simulink model "lht_workflow"  (R2020a)
settings: Solver=FixedStepDiscrete  StartTime=0.0  StopTime=inf  RelTol=1e-3
InitFcn:
  | % Clear workspace
  | clc; clear; close all;
  | 
  | % Set parameters
  | height = 240;
  | width = 320;
  | sobelThreshold = 30;
  | dTheta = 1;
  | dRho = 1;
  | 
  | % Read in image and resize
  | I = imread('roof.bmp');
  | Ir = imresize(I, [height, width]);
  | 
  | % Get greyscale
  | Y = rgb2gray(Ir);
  | 
  | % Get Edge and Gradient Orientation image
  | [edge] = Sobel(Y, sobelThreshold);
  | 
  | % Create input array
  | inarray = uint8(fi(edge, 0, 1, 0));
  | 
  | hdlset_param(gcs, 'GenerateValidationModel', 'on');
  | 
  | % Memory
  | maxRho = ceil(sqrt((height/2)^2+(width/2)^2));
  | bitsRho = ceil(log2(maxRho*2));
StopFcn:
  | %Get theta and rho
  | theta = 0:dTheta:180-dTheta;
  | 
  | A = reshape(out.simout, [maxRho*2, numel(theta)]);
  | 
  | plot3DHPS(A);
libraries: hdlsllib x5, simulink x2, dspsrcs4 x1
settings Model: DataTypeOverride=Off  SimulationMode=accelerator  Creator=david  LastModifiedBy=david
settings DataIOCC: SaveOutput=off  SaveTime=off
settings OptimizationCC: BlockReduction=off  ConditionallyExecuteInputs=off  DefaultParameterBehavior=Inlined
settings DebuggingCC: AlgebraicLoopMsg=error  SingleTaskRateTransMsg=error
settings HardwareCC: ProdBitPerPointer=32  ProdBitPerSizeT=32  ProdBitPerPtrDiffT=32  ProdLargestAtomicFloat=None  ProdIntDivRoundTo=Undefined  ProdEndianess=Unspecified  ProdWordSize=32  ProdHWDeviceType=ASIC/FPGA->ASIC/FPGA  TargetBitPerPointer=64  TargetBitPerSizeT=64  TargetBitPerPtrDiffT=64  TargetLongLongMode=on  TargetIntDivRoundTo=Zero  TargetEndianess=LittleEndian  TargetWordSize=64  TargetHWDeviceType=Custom Processor->MATLAB Host Computer  ProdEqTarget=off
settings SFSimCC: CustomCodeUndefinedFunction=UseInterfaceOnly

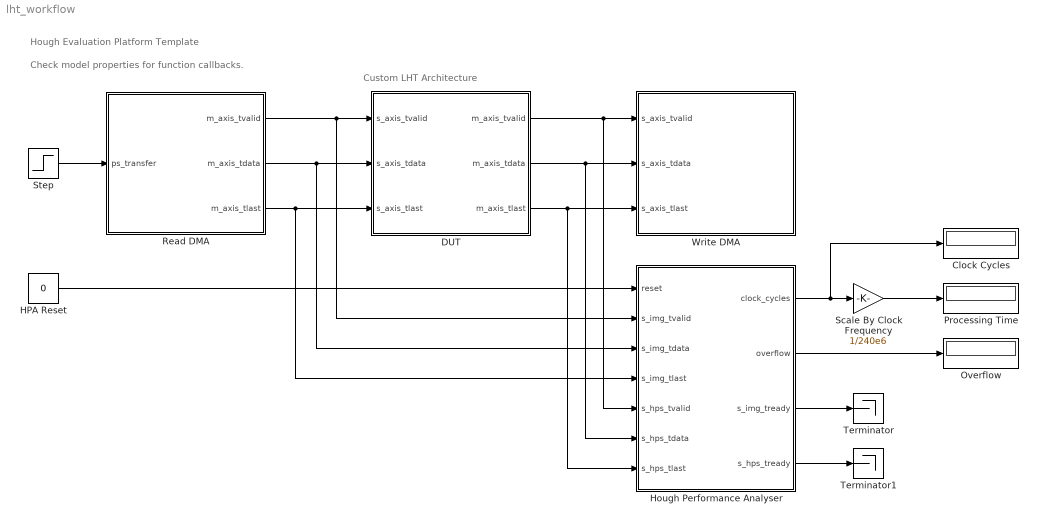
== system lht_workflow ==
  note: Custom LHT Architecture
  note: Check model properties for function callbacks.
  note: Hough Evaluation Platform Template
  Clock Cycles : Display
  DUT : Subsystem  TreatAsAtomicUnit=on
  HPA Reset : Constant  Value=0  OutDataTypeStr=boolean  SampleTime=1/150e6
  Hough Performance Analyser : Subsystem  TreatAsAtomicUnit=on
  Overflow : Display
  Processing Time : Display
  Read DMA : Subsystem  mask{image=inarray, clk=1/150e6}
      mask prompts: image "Input Image:"; clk "Clock Rate:"
      mask init:
      | [height, width] = size(image);
      mask DialogControl DescGroupVar Prompt: AXI-Stream Image Input
      mask DialogControl DescTextVar Prompt: This block simulates an AXI-Stream image input for interfacing to a hardware accelerator or IP Core.
      mask DialogControl ParameterGroupVar Prompt: Main
  Scale By Clock Frequency : Gain  Gain=1/240e6  ParamDataTypeStr=double  OutDataTypeStr=double
  Step : Step  Time=2/150e6  SampleTime=1/150e6
  Terminator : Terminator
  Terminator1 : Terminator
  Write DMA : Subsystem  mask{height=ceil(sqrt((height/2)^2+(width/2)^2))*2, width=numel([0:1:179]), clk=1/150e6, d=0}
      mask prompts: height "Image Height:"; width "Image Width:"; clk "Clock Rate:"; d "Frame Capture Number"
      mask DialogControl DescGroupVar Prompt: AXI-Stream Image Output
      mask DialogControl DescTextVar Prompt: Image output using the AXI-Stream interface. Simulates an AXI DMA write channel.
      mask DialogControl ParameterGroupVar Prompt: Main
  wires:
  Hough Performance Analyser/3(s_img_tready) -> Terminator/1
  Hough Performance Analyser/4(s_hps_tready) -> Terminator1/1
  Step/1 -> Read DMA/1(ps_transfer)
  HPA Reset/1 -> Hough Performance Analyser/1(reset)
  Hough Performance Analyser/2(overflow) -> Overflow/1
  Read DMA/2(m_axis_tdata) -> DUT/2(s_axis_tdata), Hough Performance Analyser/3(s_img_tdata)
  Read DMA/1(m_axis_tvalid) -> DUT/1(s_axis_tvalid), Hough Performance Analyser/2(s_img_tvalid)
  Read DMA/3(m_axis_tlast) -> DUT/3(s_axis_tlast), Hough Performance Analyser/4(s_img_tlast)
  DUT/1(m_axis_tvalid) -> Write DMA/1(s_axis_tvalid), Hough Performance Analyser/5(s_hps_tvalid)
  DUT/2(m_axis_tdata) -> Write DMA/2(s_axis_tdata), Hough Performance Analyser/6(s_hps_tdata)
  DUT/3(m_axis_tlast) -> Write DMA/3(s_axis_tlast), Hough Performance Analyser/7(s_hps_tlast)
  Scale By Clock Frequency/1 -> Processing Time/1
  Hough Performance Analyser/1(clock_cycles) -> Scale By Clock Frequency/1, Clock Cycles/1

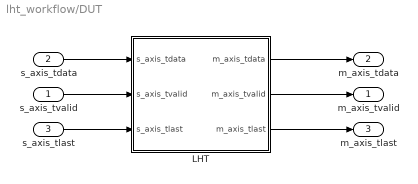
== system lht_workflow/DUT ==
  s_axis_tvalid : Inport
  s_axis_tdata : Inport  Port=2
  s_axis_tlast : Inport  Port=3
  LHT : Subsystem
  m_axis_tvalid : Outport  VectorParamsAs1DForOutWhenUnconnected=off
  m_axis_tdata : Outport  Port=2  VectorParamsAs1DForOutWhenUnconnected=off
  m_axis_tlast : Outport  Port=3  VectorParamsAs1DForOutWhenUnconnected=off
  wires:
  LHT/2(m_axis_tvalid) -> m_axis_tvalid/1
  LHT/1(m_axis_tdata) -> m_axis_tdata/1
  LHT/3(m_axis_tlast) -> m_axis_tlast/1
  s_axis_tlast/1 -> LHT/3(s_axis_tlast)
  s_axis_tvalid/1 -> LHT/2(s_axis_tvalid)
  s_axis_tdata/1 -> LHT/1(s_axis_tdata)

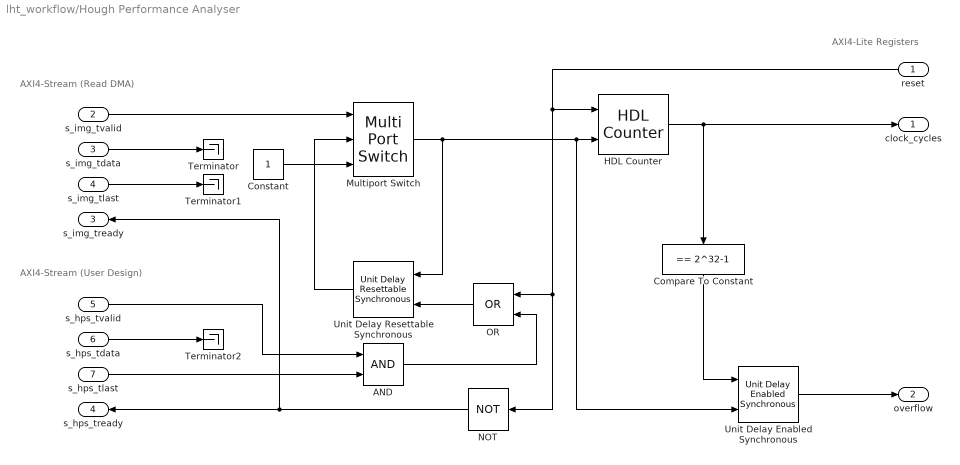
== system lht_workflow/Hough Performance Analyser ==
  note: AXI4-Lite Registers
  note: AXI4-Stream (User Design)
  note: AXI4-Stream (Read DMA)
  reset : Inport
  s_img_tvalid : Inport  Port=2
  s_img_tdata : Inport  Port=3
  s_img_tlast : Inport  Port=4
  s_hps_tvalid : Inport  Port=5
  s_hps_tdata : Inport  Port=6
  s_hps_tlast : Inport  Port=7
  AND : Logic  IconShape=distinctive  AllPortsSameDT=off  OutDataTypeStr=boolean
  Compare To Constant : simulink/Logic and Bit Operations/Compare To Constant  relop===  const=2^32-1  OutDataTypeStr=boolean
  Constant : Constant  OutDataTypeStr=boolean  SampleTime=-1
  HDL Counter : hdlsllib/Sources/HDL Counter  CountType=Count limited  CountInit=0  CountStep=1  CountMax=2^32-1  CountFromType=Initial value  CountFrom=0  CountResetPort=on  CountLoadPort=off  CountEnbPort=on  CountDirPort=off  CountDataType=Unsigned  CountWordLen=32  CountFracLen=0  CountSampTime=1
  Multiport Switch : MultiPortSwitch  DataPortOrder=Zero-based contiguous  Inputs=2  zeroidx=on
  NOT : Logic  Operator=NOT  IconShape=distinctive  AllPortsSameDT=off  OutDataTypeStr=boolean
  OR : Logic  Operator=OR  IconShape=distinctive  AllPortsSameDT=off  OutDataTypeStr=boolean
  Terminator : Terminator
  Terminator1 : Terminator
  Terminator2 : Terminator
  Unit Delay Enabled Synchronous : hdlsllib/Discrete/Unit Delay Enabled Synchronous  InitialCondition=0.0  SampleTime=-1
      settings: SourceProductBaseCode=SL
  Unit Delay Resettable Synchronous : hdlsllib/Discrete/Unit Delay Resettable Synchronous  InitialCondition=0.0  SampleTime=-1
      settings: SourceProductBaseCode=SL
  clock_cycles : Outport
  overflow : Outport  Port=2
  s_img_tready : Outport  Port=3
  s_hps_tready : Outport  Port=4
  wires:
  Constant/1 -> Multiport Switch/3
  Unit Delay Resettable Synchronous/1 -> Multiport Switch/2
  Multiport Switch/1 -> Unit Delay Resettable Synchronous/1, Unit Delay Enabled Synchronous/2, HDL Counter/2
  Compare To Constant/1 -> Unit Delay Enabled Synchronous/1
  Unit Delay Enabled Synchronous/1 -> overflow/1
  HDL Counter/1 -> Compare To Constant/1, clock_cycles/1
  s_hps_tdata/1 -> Terminator2/1
  s_img_tdata/1 -> Terminator/1
  reset/1 -> NOT/1, OR/1, HDL Counter/1
  s_img_tlast/1 -> Terminator1/1
  OR/1 -> Unit Delay Resettable Synchronous/2
  s_img_tvalid/1 -> Multiport Switch/1
  AND/1 -> OR/2
  s_hps_tlast/1 -> AND/2
  s_hps_tvalid/1 -> AND/1
  NOT/1 -> s_img_tready/1, s_hps_tready/1

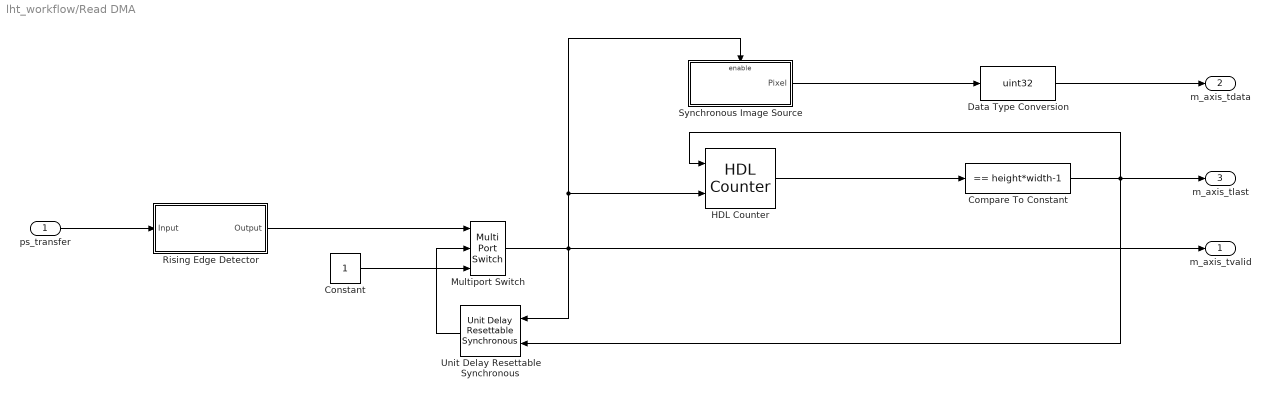
== system lht_workflow/Read DMA ==
  ps_transfer : Inport
  Compare To Constant : simulink/Logic and Bit Operations/Compare To Constant  relop===  const=height*width-1  OutDataTypeStr=boolean
  Constant : Constant  OutDataTypeStr=boolean  SampleTime=-1
  Data Type Conversion : DataTypeConversion  OutDataTypeStr=uint32
  HDL Counter : hdlsllib/Sources/HDL Counter  CountType=Free running  CountInit=0  CountStep=1  CountMax=width*height-1  CountFromType=Initial value  CountFrom=0  CountResetPort=on  CountLoadPort=off  CountEnbPort=on  CountDirPort=off  CountDataType=Unsigned  CountWordLen=32  CountFracLen=0  CountSampTime=1
  Multiport Switch : MultiPortSwitch  DataPortOrder=Zero-based contiguous  Inputs=2  zeroidx=on
  Rising Edge Detector : Subsystem
  Synchronous Image Source : Subsystem
  Unit Delay Resettable Synchronous : hdlsllib/Discrete/Unit Delay Resettable Synchronous  InitialCondition=0.0  SampleTime=-1
      settings: SourceProductBaseCode=SL
  m_axis_tvalid : Outport
  m_axis_tdata : Outport  Port=2
  m_axis_tlast : Outport  Port=3
  wires:
  HDL Counter/1 -> Compare To Constant/1
  Synchronous Image Source/1(Pixel) -> Data Type Conversion/1
  Multiport Switch/1 -> Unit Delay Resettable Synchronous/1, HDL Counter/2, Synchronous Image Source/Enable, m_axis_tvalid/1
  Compare To Constant/1 -> Unit Delay Resettable Synchronous/2, HDL Counter/1, m_axis_tlast/1
  Data Type Conversion/1 -> m_axis_tdata/1
  ps_transfer/1 -> Rising Edge Detector/1(Input)
  Unit Delay Resettable Synchronous/1 -> Multiport Switch/2
  Rising Edge Detector/1(Output) -> Multiport Switch/1
  Constant/1 -> Multiport Switch/3

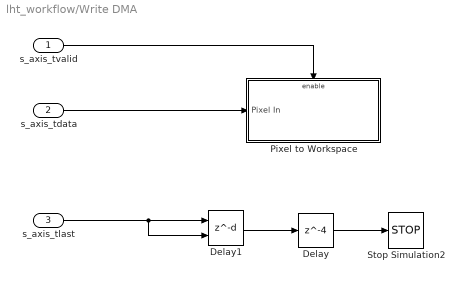
== system lht_workflow/Write DMA ==
  s_axis_tvalid : Inport
  s_axis_tdata : Inport  Port=2
  s_axis_tlast : Inport  Port=3
  Delay : Delay  DelayLength=4
  Delay1 : Delay  DelayLength=d  ShowEnablePort=on
      settings: InputPortMap=u0,e6
  Pixel to Workspace : Subsystem
  Stop Simulation2 : Stop
  wires:
  s_axis_tvalid/1 -> Pixel to Workspace/Enable
  s_axis_tdata/1 -> Pixel to Workspace/1(Pixel In)
  s_axis_tlast/1 -> Delay1/2, Delay1/1
  Delay1/1 -> Delay/1
  Delay/1 -> Stop Simulation2/1

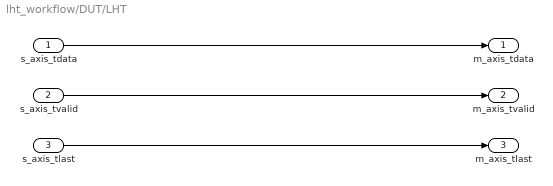
== system lht_workflow/DUT/LHT ==
  s_axis_tdata : Inport
  s_axis_tvalid : Inport  Port=2
  s_axis_tlast : Inport  Port=3
  m_axis_tdata : Outport  VectorParamsAs1DForOutWhenUnconnected=off
  m_axis_tvalid : Outport  Port=2  VectorParamsAs1DForOutWhenUnconnected=off
  m_axis_tlast : Outport  Port=3  VectorParamsAs1DForOutWhenUnconnected=off
  wires:
  s_axis_tdata/1 -> m_axis_tdata/1
  s_axis_tvalid/1 -> m_axis_tvalid/1
  s_axis_tlast/1 -> m_axis_tlast/1

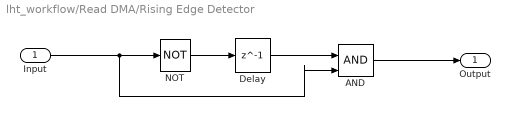
== system lht_workflow/Read DMA/Rising Edge Detector ==
  Input : Inport
  AND : Logic  IconShape=distinctive  AllPortsSameDT=off  OutDataTypeStr=boolean
  Delay : Delay  DelayLength=1
  NOT : Logic  Operator=NOT  IconShape=distinctive  AllPortsSameDT=off  OutDataTypeStr=boolean
  Output : Outport  VectorParamsAs1DForOutWhenUnconnected=off
  wires:
  NOT/1 -> Delay/1
  Input/1 -> AND/2, NOT/1
  Delay/1 -> AND/1
  AND/1 -> Output/1

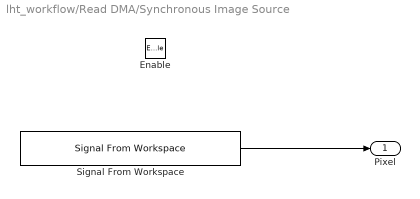
== system lht_workflow/Read DMA/Synchronous Image Source ==
  Enable : EnablePort
  Signal From Workspace : dspsrcs4/Signal From Workspace  X=reshape(image', [height*width, 1])  Ts=clk  nsamps=1  OutputAfterFinalValue=Cyclic repetition  ignoreOrWarnInputAndFrameLengths=off  OutputFrames=off
  Pixel : Outport
  wires:
  Signal From Workspace/1 -> Pixel/1

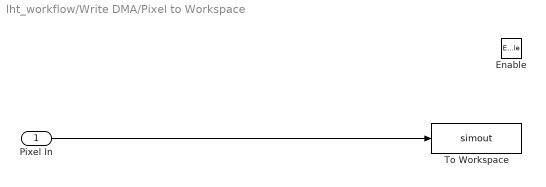
== system lht_workflow/Write DMA/Pixel to Workspace ==
  Pixel In : Inport
  Enable : EnablePort
  To Workspace : ToWorkspace  VariableName=simout  SampleTime=-1
      settings: MaxDataPoints=height*width  Save2DSignal=2-D array (concatenate along first dimension)
  wires:
  Pixel In/1 -> To Workspace/1
